simulink model "Sampling"  (R2023a)
settings: Solver=VariableStepAuto  StartTime=0.0  StopTime=10.0  RelTol=1e-3
libraries: simulink x1, dspsigops x1
settings Model: Creator=ADMIN  LastModifiedBy=ADMIN

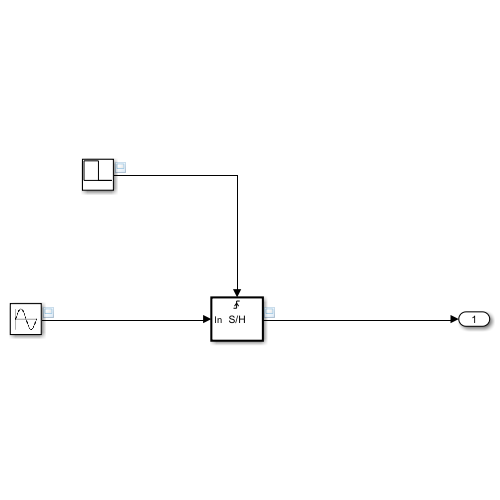
[thumbnail: Simulink's stored preview of the top-level diagram]
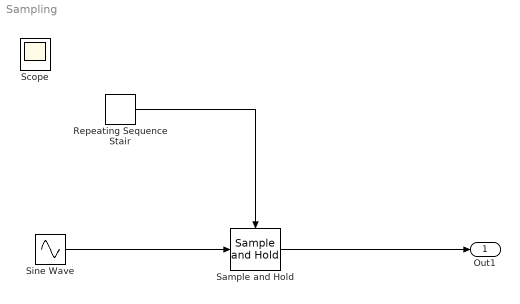
== system Sampling ==
  Repeating Sequence Stair : simulink/Sources/Repeating Sequence Stair  OutValues=[1 0].'  tsamp=-1  OutMin=[]  OutMax=[]  OutDataTypeStr=double  OutputDataTypeScalingMode=double  OutDataType=fixdt(0,8)  ConRadixGroup=Best Precision: Vector-wise  OutScaling=2^-12
  Sample and Hold : dspsigops/Sample and Hold  trig=Rising edge  initCond=0  latchinput=off
  Sine Wave : Sin  Amplitude=5  SampleTime=0
  Out1 : Outport
  Scope : Scope
  wires:
  Sample and Hold/1 -> Out1/1
  Repeating Sequence Stair/1 -> Sample and Hold/Trigger
  Sine Wave/1 -> Sample and Hold/1
